simulink model "control_input"  (Simulink 7.5)
settings: Solver=FixedStepDiscrete  StartTime=0.0  StopTime=10.0  FixedStep=SampleTime  RelTol=1e-3
undefined symbols (not defined in the file or in its folder): SampleTime
libraries: simulink x1
settings Model: Creator=austinmurch  LastModifiedBy=Andrei
settings OptimizationCC: InlineParams=on  SimCompilerOptimization=On
settings DebuggingCC: StrictBusMsg=Warning
settings HardwareCC: ProdIntDivRoundTo=Zero  ProdEndianess=BigEndian  ProdHWDeviceType=Freescale->32-bit PowerPC

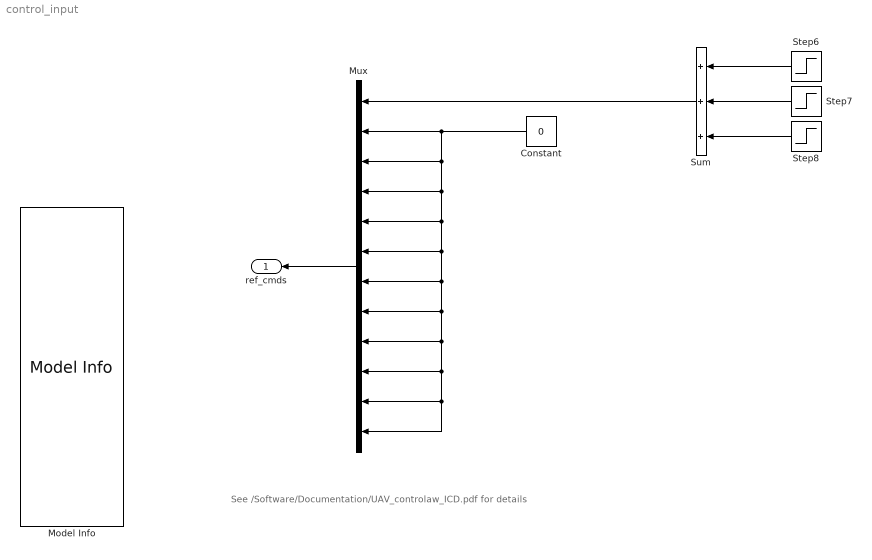
== system control_input ==
  note: See /Software/Documentation/UAV_controlaw_ICD.pdf
      | for details
  Constant : Constant  Value=0  OutDataType=fixdt(1, 16)  OutScaling=2^0
  Model Info : simulink/Model-Wide Utilities/Model Info  SystemSampleTime=-1  InitialBlockCM=None  BlockCM=None  Frame=on  DisplayStringWithTags=|  HorizontalTextAlignment=Center  LeftAlignmentValue=0.5  SourceBlockDiagram=control_input  TagMaxNumber=20
      | Ref Cmd Port Info
      | 
      | 1. phi_cmd
      | 2. theta_cmd
      | 3. psi_cmd
      | 4. p_cmd
      | 5. q_cmd
      | 6. r_cmd
      | 7. V_s_cmd
      | 8. h_cmd
      | 9. gndtrk_cmd
      | 10. aoa_cmd
      | 11. aos_cmd
      | 12. gamma_cmd
  Mux : Mux  Inputs=12
  Step6 : Step  After=5*pi/180  SampleTime=SampleTime
  Step7 : Step  Time=5  After=-10*pi/180  SampleTime=SampleTime
  Step8 : Step  Time=9  After=5*pi/180  SampleTime=SampleTime
  Sum : Sum  Inputs=+++  SampleTime=SampleTime
  ref_cmds : Outport
  wires:
  Mux/1 -> ref_cmds/1
  Step6/1 -> Sum/1
  Step7/1 -> Sum/2
  Step8/1 -> Sum/3
  Sum/1 -> Mux/1
  Constant/1 -> Mux/2, Mux/3, Mux/4, Mux/5, Mux/6, Mux/7, Mux/8, Mux/9, Mux/10, Mux/11, Mux/12
